simulink model "lab6"  (R2022a)
settings: Solver=FixedStepAuto  StartTime=0.0  StopTime=3  FixedStep=1e-6  MaxStep=1e-5  RelTol=1e-5  EnableMultiTasking=on
undefined symbols (not defined in the file): f_e, I_n, J, km, Lr, Ls, m_f, Pn, Rr, Rs, T_e_rated, T_me_load, U_s, w_ref, zp
libraries: simulink x9, spsFourierLib x6, spsControlledVoltageSourceLib x3, spsAsynchronousMachineSIUnitsLib x2, spsSeriesRLCBranchLib x2, spsThreePhaseVIMeasurementLib x2, spsVoltageMeasurementLib x2, spsUniversalBridgeLib x1, spsDiodeLib x1, spsGroundLib x1, spspowerguiLib x1
settings Model: SimulationMode=accelerator  Creator=Trant  LastModifiedBy=81502
settings SolverCC: AlgebraicLoopSolver=TrustRegion
settings DataIOCC: ReturnWorkspaceOutputs=off
settings DebuggingCC: UnconnectedInputMsg=warning  UnconnectedOutputMsg=warning  UnconnectedLineMsg=warning  SFExecutionAtInitializationDiag=none  SFMachineParentedDataDiag=warning  ArithmeticOperatorsInVariantConditions=warning
settings SFSimCC: SimUseLocalCustomCode=off  CustomCodeUndefinedFunction=UseInterfaceOnly
settings RTWCC: RTWUseLocalCustomCode=off  DLArmComputeVersion=19.05
settings CodeAppCC: StateflowObjectComments=on
settings ConfigComp: CovMetricSettings=dw  CovSaveCumulativeToWorkspaceVar=on  CovSaveSingleToWorkspaceVar=on  CovExternalEMLEnable=off
settings SimscapeCC: SimscapeNormalizeSystem=off

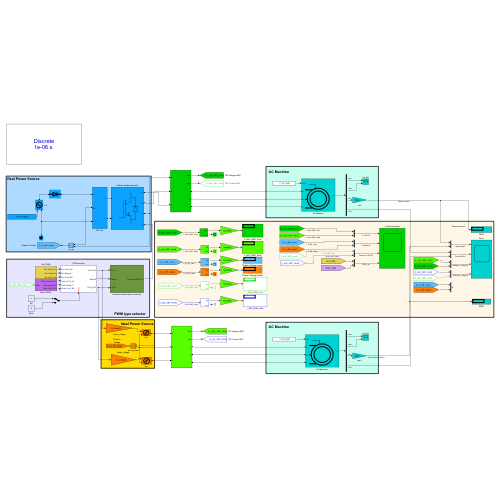
[thumbnail: Simulink's stored preview of the top-level diagram]
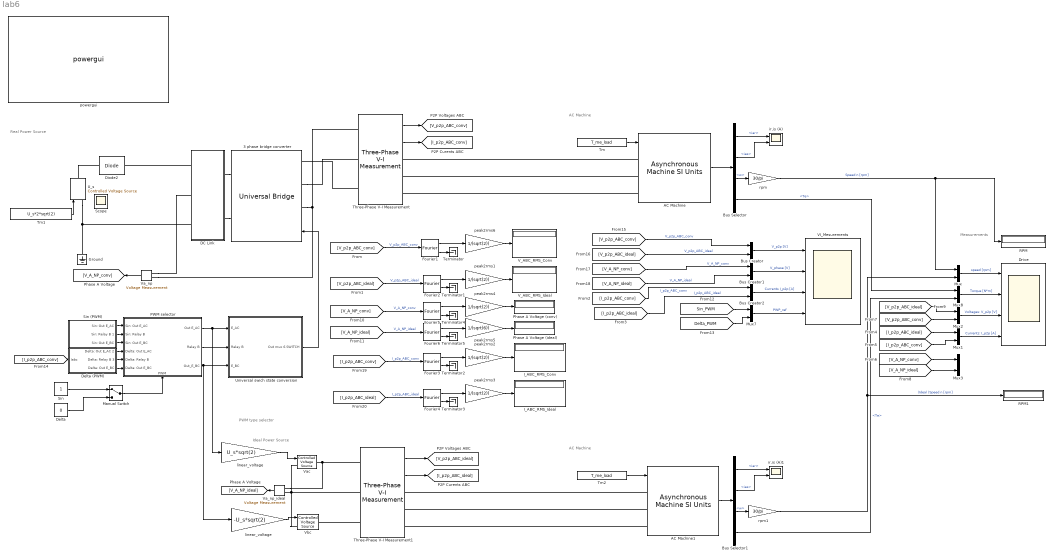
== system lab6 ==
  note: Measurements
  note: Ideal Power Source
  note: Real Power Source
  note: PWM type selector
  note: AC Machine
  note: AC Machine
  3 phase bridge converter : spsUniversalBridgeLib/Universal Bridge  Arms=3  SnubberResistance=1e5  SnubberCapacitance=inf  Device=IGBT / Diodes  Ron=1e-2  Lon=0  ForwardVoltages="[  1.5  0.7  ]"  ForwardVoltage=0  GTOparameters=[ 10e-6 , 20e-6 ]  IGBTparameters=[ 1e-6 , 2e-6 ]  Measurements=None  Measurements_2=None  converterType=Rectifier
  AC Machine : spsAsynchronousMachineSIUnitsLib/Asynchronous Machine SI Units  RotorType=Squirrel-cage  PresetModel=No  MechanicalLoad=Torque Tm  ShowDetailedParameters=on  ReferenceFrame=Stationary  Units=SI  MeasurementBus=on  NominalParameters=[ Pn, U_s*sqrt(3), f_e ]  VoltageRatio=1  Stator="[ Rs  Ls ]"  Rotor="[Rr  Lr ]"  Cage1=[ 0.022 0.226/377]  Cage2=[ 0.022 0.226/377]  Lm=Lm  Mechanical="[ J  0 zp]"  PolePairs=2  InitialConditions="[ 1,0   0,0,0   0,0,0 ]"  SimulateSaturation=off  Saturation=[14.03593122, 27.81365428, 53.79336849, 72.68890987, 97.98006896, 148.6815601, 215.7428561, 302.9841135, 428.7778367 ; 230, 322, 414, 460, 506, 552, 598, 644, 690]  LoadFlowParameters=0  TsPowergui=0  TsBlock=-1  IterativeModel=Trapezoidal non iterative  IterativeDiscreteModel=Trapezoidal non iterative  Pmec=0
      settings: AttributesFormatString=\n
  AC Machine1 : spsAsynchronousMachineSIUnitsLib/Asynchronous Machine SI Units  RotorType=Squirrel-cage  PresetModel=No  MechanicalLoad=Torque Tm  ShowDetailedParameters=on  ReferenceFrame=Stationary  Units=SI  MeasurementBus=on  NominalParameters=[ Pn, U_s*sqrt(3), f_e ]  VoltageRatio=1  Stator="[ Rs  Ls ]"  Rotor="[Rr  Lr ]"  Cage1=[ 0.022 0.226/377]  Cage2=[ 0.022 0.226/377]  Lm=Lm  Mechanical="[ J  0 zp]"  PolePairs=2  InitialConditions="[ 1,0   0,0,0   0,0,0 ]"  SimulateSaturation=off  Saturation=[14.03593122, 27.81365428, 53.79336849, 72.68890987, 97.98006896, 148.6815601, 215.7428561, 302.9841135, 428.7778367 ; 230, 322, 414, 460, 506, 552, 598, 644, 690]  LoadFlowParameters=0  TsPowergui=0  TsBlock=-1  IterativeModel=Trapezoidal non iterative  IterativeDiscreteModel=Trapezoidal non iterative  Pmec=0
      settings: AttributesFormatString=\n
  Bus Creator : BusCreator  Inputs=2
  Bus Creator1 : BusCreator  Inputs=2
  Bus Creator2 : BusCreator  Inputs=2
  Bus Selector : BusSelector  OutputSignals=iar,ias,w,Te
  Bus Selector1 : BusSelector  OutputSignals=iar,ias,w,Te
  DC Link : Subsystem
  Delta : Constant  Value=0
  "Delta (PWM) " : Subsystem
  Diode2 : spsDiodeLib/Diode  Ron=0.0000001  Lon=0  Vf=0.0000001  IC=0  UseSnubber=0  Rs=inf  Cs=250e-9  Measurements=off
  Drive : Scope  NumInputPorts=4
  Fourier{1..6} (6 alike) : spsFourierLib/Fourier  Freq=f_e  n=1  InInit=[0, 0]  Ts=0
      settings: SourceProductBaseCode=PS
  Ground : spsGroundLib/Ground  LConnTagsString=a
  I_ABC_RMS_Conv : Display
      settings: Decimation=100
  I_ABC_RMS_Ideal : Display
      settings: Decimation=100
  Manual Switch : ManualSwitch
  Mux{,1..3,7..8} (6 alike) : Mux  Inputs=2
  PWM selector : Subsystem
      settings: PortSchema="{\"entries\":[{\"content\":{\"sides\":[{\"content\":{\"connectorIds\":[\"In1\",\"In2\",\"In3\",\"In4\",\"In5\",\"In6\"]},\"type\":\"ConnectorPlacement.EquallySpacedRectSide\",\"uuid\":\"d8825297-29c5-47ea-8460-276057c08024\"},{\"content\":{\"connectorIds\":[\"Out1\",\"Out2\",\"Out3\"],\"side\":\"RIGHT\"},\"type\":\"ConnectorPlacement.EquallySpacedRectSide\",\"uuid\":\"df0a2572-9195-4f57-b13e-7b5fffdd47ce\"},{\"content\":{\"connectorIds\":[],\"side\":\"TOP\"},\"type\":\"ConnectorPlacement.EquallySpacedRectSide\",\"uuid\":\"3bcfb922-02d6-49ee-9ecc-d9568c4dbca9\"},{\"content\":{\"connectorIds\":[\"In7\"],\"side\":\"BOTTOM\"},\"type\":\"ConnectorPlacement.EquallySpacedRectSide\",\"uuid\":\"29fdab77-a4c0-4546-9e45-02849de3b5bd\"},{\"content\":{\"connectorIds\":[],\"side\":\"HIDDEN\"},\"type\":\"ConnectorPlacement.EquallySpacedRectSide\",\"uuid\":\"147cb719-0326-42c1-9162-cd1cd750ef12\"}]},\"type\":\"ConnectorPlacement.EquallySpacedConnector\",\"uuid\":\"5ed61148-1717-428a-bdaf-bb7d5a590e8d\"}],\"packageUris\":[\"http://schema.mathworks.com/mf0/Connector/R2020b\"],\"version\":\"1.0\"}"
  Phase A Voltage (conv) : Display
      settings: Decimation=100
  Phase A Voltage (ideal) : Display
      settings: Decimation=100
  RPM : Display
      settings: Decimation=100
  RPM1 : Display
      settings: Decimation=100
  Sin : Constant
  Sin (PWM) : Subsystem
  Terminator{,1..5} (6 alike) : Terminator
  Three-Phase V-I Measurement : spsThreePhaseVIMeasurementLib/Three-Phase V-I Measurement  VoltageMeasurement=phase-to-phase  SetLabelV=off  LabelV=Vabc  Vpu=off  VpuLL=off  CurrentMeasurement=yes  SetLabelI=off  LabelI=Iabc  Ipu=off  Pbase=100e6  Vbase=500e3  OutputType=Complex  PhasorSimulation=off  PSBequivalent=0
  Three-Phase V-I Measurement1 : spsThreePhaseVIMeasurementLib/Three-Phase V-I Measurement  VoltageMeasurement=phase-to-phase  SetLabelV=off  LabelV=Vabc  Vpu=off  VpuLL=off  CurrentMeasurement=yes  SetLabelI=off  LabelI=Iabc  Ipu=off  Pbase=100e6  Vbase=500e3  OutputType=Complex  PhasorSimulation=off  PSBequivalent=0
  Tm : Constant  Value=T_me_load
  Tm1 : Constant  Value=U_s*2*sqrt(2)  VectorParams1D=off
  Tm2 : Constant  Value=T_me_load
  U_s : spsControlledVoltageSourceLib/Controlled Voltage Source  Description=source block  Initialize=on  Source_Type=AC  Amplitude=0  Phase=0  Frequency=0  Measurements=None
      settings: AttributesFormatString=\n
  Universal swich state conversion : Subsystem
  VI_Mesurements : Scope  NumInputPorts=4
  V_ABC_RMS_Conv : Display
      settings: Decimation=100
  V_ABC_RMS_Ideal : Display
      settings: Decimation=100
  Va_np : spsVoltageMeasurementLib/Voltage Measurement  Tag=PoWeRsYsTeMmEaSuReMeNt  PhasorSimulation=off  OutputType=Magnitude  PSBequivalent=0
  Va_np_ideal : spsVoltageMeasurementLib/Voltage Measurement  Tag=PoWeRsYsTeMmEaSuReMeNt  PhasorSimulation=off  OutputType=Magnitude  PSBequivalent=0
  Vac : spsControlledVoltageSourceLib/Controlled Voltage Source  Description=source block  Initialize=on  Source_Type=AC  Amplitude=0  Phase=0  Frequency=0  Measurements=None
      settings: AttributesFormatString=\n
  "Vbc " : spsControlledVoltageSourceLib/Controlled Voltage Source  Description=source block  Initialize=on  Source_Type=AC  Amplitude=0  Phase=0  Frequency=0  Measurements=None
      settings: AttributesFormatString=\n
  ir,is (A) : Scope  NumInputPorts=2
  ir,is (A)1 : Scope  NumInputPorts=2
  linear_voltage : Gain  Gain=U_s*sqrt(2)  SaturateOnIntegerOverflow=on  OutDataTypeStr=Inherit: Same as input  ParamDataTypeStr=Inherit: Same as input
  "linear_voltage " : Gain  Gain=-U_s*sqrt(2)  SaturateOnIntegerOverflow=on  OutDataTypeStr=Inherit: Same as input  ParamDataTypeStr=Inherit: Same as input
  peak2rms{1..4,6} (5 alike) : Gain  Gain=1/(sqrt(2))  SaturateOnIntegerOverflow=on  OutDataTypeStr=Inherit: Same as input  ParamDataTypeStr=Inherit: Same as input
  peak2rms5 : Gain  Gain=1/(sqrt(6))  SaturateOnIntegerOverflow=on  OutDataTypeStr=Inherit: Same as input  ParamDataTypeStr=Inherit: Same as input
  powergui : spspowerguiLib/powergui  SimulationMode=Discrete  SampleTime=1e-6  frequency=60  Iterations=50  frequencyindice=0  Pbase=100e6  ErrMax=1e-4  UnitsV=kV  UnitsW=MW  buscounter=0  FunctionMessages=off  echomessages=off  EnableUseOfTLC=off  CurrentSourceSwitches=on  DisableSnubberDevices=off  DisableRonSwitches=off  DisableVfSwitches=off  DisplayEquations=off  AutomaticDiscreteSolvers=off  SolverType=Tustin/Backward Euler (TBE)  Interpol=off  ExternalGateDelay=off  methode=off  Ts=100  x0status=blocks  SPID=off  SwTol=0  HookPort=off  NonlinearTolerance=1e-4  nMaxIteration=100  ContinueOnMaxIteration=off  RestoreLinks=warning  ResistiveCurrentMeasurement=off  Frange=[0:2:500]  Ylog=off  Xlog=on  ShowGrid=off  save=off  variable=ZData  structure=VI_mesurements  ZoomFFT=off  StartTime=1.55  cycles=1  DisplayStyle=1  fundamental=50  FreqAxis=on  MaxFrequency=40000  frequencyindicesteady=1  RmsSteady=1  display=off
  rpm : Gain  Gain=30/pi  SaturateOnIntegerOverflow=on  OutDataTypeStr=Inherit: Same as input  ParamDataTypeStr=Inherit: Same as input
  rpm1 : Gain  Gain=30/pi  SaturateOnIntegerOverflow=on  OutDataTypeStr=Inherit: Same as input  ParamDataTypeStr=Inherit: Same as input
  Scope : Scope
  wires:
  Tm/1 -> AC Machine/1
  Bus Selector/3 -> rpm/1  "<w>"
  Fourier1/2 -> Terminator/1
  rpm/1 -> Mux/1, RPM/1  "Speed n [rpm]"
  Bus Selector/2 -> ir,is (A)/2  "<ias>"
  peak2rms6/1 -> V_ABC_RMS_Conv/1
  Bus Selector/1 -> ir,is (A)/1  "<iar>"
  AC Machine/1 -> Bus Selector/1
  Fourier1/1 -> peak2rms6/1
  Tm1/1 -> U_s/1
  "linear_voltage "/1 -> "Vbc "/1
  linear_voltage/1 -> Vac/1
  Fourier2/1 -> peak2rms1/1
  Fourier2/2 -> Terminator1/1
  peak2rms1/1 -> V_ABC_RMS_Ideal/1
  Universal swich state conversion/1(Out mux 6 SWITCH) -> 3 phase bridge converter/1
  Manual Switch/1 -> PWM selector/7(PWM)
  Sin/1 -> Manual Switch/1
  Delta/1 -> Manual Switch/2
  Sin (PWM)/1("Sin: Out E_AC ") -> PWM selector/1(Sin: Out E_AC)
  Sin (PWM)/2(Sin: Relay B 1) -> PWM selector/2(Sin: Relay B)
  Sin (PWM)/3(Sin: Out E_BC) -> PWM selector/3(Sin: Out E_BC)
  "Delta (PWM) "/1(Delta: Out E_AC 2) -> PWM selector/4(Delta: Out E_AC)
  "Delta (PWM) "/2(Delta: Relay B 3) -> PWM selector/5(Delta: Relay B)
  "Delta (PWM) "/3(Delta: Out E_BC) -> PWM selector/6(Delta: Out E_BC)
  PWM selector/3(Out_E_BC) -> "linear_voltage "/1, Universal swich state conversion/3(E_BC)
  PWM selector/2(Relay B) -> Universal swich state conversion/2("Relay B ")
  PWM selector/1(Out E_AC) -> Universal swich state conversion/1("E_AC "), linear_voltage/1
  Three-Phase V-I Measurement/1 -> [V_p2p_ABC_conv]
  Three-Phase V-I Measurement1/1 -> [V_p2p_ABC_ideal]
  Three-Phase V-I Measurement1/2 -> [I_p2p_ABC_ideal]
  Three-Phase V-I Measurement/2 -> [I_p2p_ABC_conv]
  [V_p2p_ABC_conv] -> Fourier1/1  "V_p2p_ABC_conv"
  [V_p2p_ABC_ideal] -> Fourier2/1  "V_p2p_ABC_ideal"
  AC Machine1/1 -> Bus Selector1/1
  Tm2/1 -> AC Machine1/1
  Bus Selector1/2 -> ir,is (A)1/2  "<ias>"
  Bus Selector1/1 -> ir,is (A)1/1  "<iar>"
  rpm1/1 -> RPM1/1, Mux/2  "(Ideal )Speed n [rpm]"
  Bus Selector1/3 -> rpm1/1  "<w>"
  Mux/1 -> Drive/1  "speed [rpm]"
  [I_p2p_ABC_ideal] -> Bus Creator2/2  "I_p2p_ABC_ideal"
  [I_p2p_ABC_conv] -> Bus Creator2/1  "I_p2p_ABC_conv"
  peak2rms3/1 -> I_ABC_RMS_Ideal/1
  Fourier4/2 -> Terminator3/1
  Fourier4/1 -> peak2rms3/1
  Fourier3/1 -> peak2rms2/1
  peak2rms2/1 -> I_ABC_RMS_Conv/1
  Fourier3/2 -> Terminator2/1
  [I_p2p_ABC_conv] -> Mux1/2
  [I_p2p_ABC_ideal] -> Mux1/1
  Mux1/1 -> Drive/4  "Currents: I_p2p [A]"
  [V_p2p_ABC_ideal] -> Mux2/1
  [V_p2p_ABC_conv] -> Mux2/2
  Mux2/1 -> Drive/3  "Voltages: V_p2p [V]"
  Va_np/1 -> [V_A_NP_conv]
  Va_np_ideal/1 -> [V_A_NP_ideal]
  [V_A_NP_conv] -> Fourier5/1  "V_A_NP_conv"
  Fourier5/1 -> peak2rms4/1
  peak2rms4/1 -> Phase A Voltage (conv)/1
  Fourier5/2 -> Terminator4/1
  Bus Creator/1 -> VI_Mesurements/1  "V_p2p [V]"
  Bus Creator1/1 -> VI_Mesurements/2  "V_phase [V]"
  Bus Creator2/1 -> VI_Mesurements/3  "Currents I_p2p [A]"
  [Sin_PWM] -> Mux7/1
  [Delta_PWM] -> Mux7/2
  Mux7/1 -> VI_Mesurements/4  "PWP_ref"
  [I_p2p_ABC_conv] -> "Delta (PWM) "/1("Iabc ")
  Fourier6/2 -> Terminator5/1
  peak2rms5/1 -> Phase A Voltage (ideal)/1
  Fourier6/1 -> peak2rms5/1
  Bus Selector/4 -> Mux8/1  "<Te>"
  Bus Selector1/4 -> Mux8/2  "<Te>"
  Mux8/1 -> Drive/2  "Torque [N*m]"
  [V_A_NP_conv] -> Mux3/1
  [V_A_NP_ideal] -> Mux3/2
  [V_A_NP_ideal] -> Fourier6/1  "V_A_NP_ideal"
  [V_p2p_ABC_conv] -> Bus Creator/1  "V_p2p_ABC_conv"
  [V_p2p_ABC_ideal] -> Bus Creator/2  "V_p2p_ABC_ideal"
  [V_A_NP_conv] -> Bus Creator1/1  "V_A_NP_conv"
  [V_A_NP_ideal] -> Bus Creator1/2  "V_A_NP_ideal"
  [I_p2p_ABC_ideal] -> Fourier4/1  "I_p2p_ABC_ideal"
  [I_p2p_ABC_conv] -> Fourier3/1  "I_p2p_ABC_conv"
  connections:
  "Vbc "/LConn1 -- Vac/LConn1 -- Va_np_ideal/LConn2 -- Three-Phase V-I Measurement1/LConn2
  Three-Phase V-I Measurement1/LConn1 -- Va_np_ideal/LConn1 -- Vac/RConn1
  AC Machine/LConn3 -- Three-Phase V-I Measurement/RConn3
  AC Machine/LConn2 -- Three-Phase V-I Measurement/RConn2
  AC Machine/LConn1 -- Three-Phase V-I Measurement/RConn1
  U_s/RConn1 -- Diode2/LConn1
  3 phase bridge converter/LConn2 -- Three-Phase V-I Measurement/LConn2
  Three-Phase V-I Measurement1/LConn3 -- "Vbc "/RConn1
  AC Machine1/LConn1 -- Three-Phase V-I Measurement1/RConn1
  AC Machine1/LConn2 -- Three-Phase V-I Measurement1/RConn2
  AC Machine1/LConn3 -- Three-Phase V-I Measurement1/RConn3
  Three-Phase V-I Measurement/LConn3 -- 3 phase bridge converter/LConn3
  3 phase bridge converter/LConn1 -- Va_np/LConn1 -- Three-Phase V-I Measurement/LConn1
  Ground/LConn1 -- U_s/LConn1 -- DC Link/LConn3
  DC Link/LConn1 -- Diode2/RConn1
  DC Link/RConn2 -- 3 phase bridge converter/RConn1
  DC Link/RConn1 -- 3 phase bridge converter/RConn2
  Va_np/LConn2 -- DC Link/LConn2

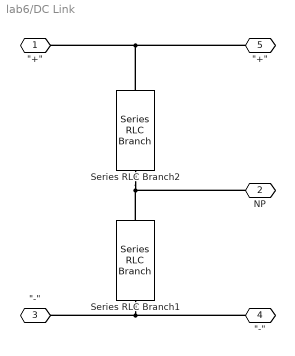
== system lab6/DC Link ==
  Series RLC Branch1 : spsSeriesRLCBranchLib/Series RLC Branch  LConnTagsString=__new0  RConnTagsString=__new0  BranchType=RC  Resistance=0.1  Inductance=1e-3  SetiL0=off  InitialCurrent=0  Capacitance=1e-3  Setx0=off  InitialVoltage=0  Measurements=None
  Series RLC Branch2 : spsSeriesRLCBranchLib/Series RLC Branch  LConnTagsString=__new0  RConnTagsString=__new0  BranchType=RC  Resistance=0.1  Inductance=1e-3  SetiL0=off  InitialCurrent=0  Capacitance=1e-3  Setx0=off  InitialVoltage=0  Measurements=None
  "\"+\"" : PMIOPort  Side=Left
  NP : PMIOPort  Port=2  Side=Left
  "\"-\"" : PMIOPort  Port=3  Side=Left
  "\"-\" " : PMIOPort  Port=4  Side=Right
  "\"+\" " : PMIOPort  Port=5  Side=Right
  connections:
  Series RLC Branch1/LConn1 -- NP/RConn1 -- Series RLC Branch2/RConn1
  Series RLC Branch1/RConn1 -- "\"-\" "/RConn1 -- "\"-\""/RConn1
  Series RLC Branch2/LConn1 -- "\"+\""/RConn1 -- "\"+\" "/RConn1

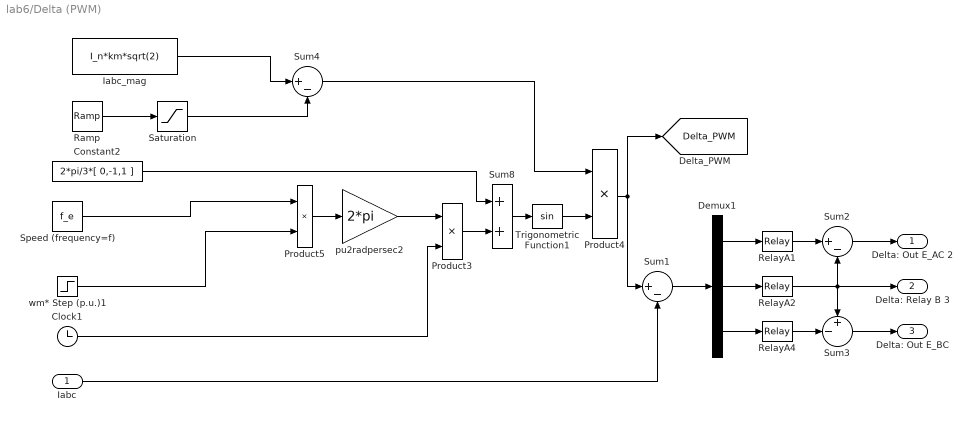
== system lab6/Delta (PWM)  ==
  "Iabc " : Inport
  Clock1 : Clock
  Constant2 : Constant  Value=2*pi/3*[ 0,-1,1 ]
  Demux1 : Demux  Outputs=3
      settings: DisplayOption=none
  Iabc_mag : Constant  Value=I_n*km*sqrt(2)
  Product3 : Product  InputSameDT=on  SaturateOnIntegerOverflow=on  OutDataTypeStr=Inherit: Same as first input
  Product4 : Product  InputSameDT=on  SaturateOnIntegerOverflow=on  OutDataTypeStr=Inherit: Same as first input
  Product5 : Product  InputSameDT=on  SaturateOnIntegerOverflow=on  OutDataTypeStr=Inherit: Same as first input
  Ramp : simulink/Sources/Ramp  slope=1  start=0  InitialOutput=0
  RelayA1 : Relay  OnSwitchValue=0.1  OffSwitchValue=-0.1
  RelayA2 : Relay  OnSwitchValue=0.1  OffSwitchValue=-0.1
  RelayA4 : Relay  OnSwitchValue=0.1  OffSwitchValue=-0.1
  Saturation : Saturate  UpperLimit=T_me_load/T_e_rated*I_n*sqrt(2)  LowerLimit=0
  Speed (frequency=f) : Constant  Value=f_e
  Sum1 : Sum  Inputs=|+-  InputSameDT=on  SaturateOnIntegerOverflow=on  OutDataTypeStr=Inherit: Same as first input
  Sum2 : Sum  Inputs=|+-  InputSameDT=on  SaturateOnIntegerOverflow=on  OutDataTypeStr=Inherit: Same as first input
  Sum3 : Sum  Inputs=+-|  InputSameDT=on  SaturateOnIntegerOverflow=on  OutDataTypeStr=Inherit: Same as first input
  Sum4 : Sum  Inputs=|+-  InputSameDT=on  SaturateOnIntegerOverflow=on  OutDataTypeStr=Inherit: Same as first input
  Sum8 : Sum  InputSameDT=on  SaturateOnIntegerOverflow=on  OutDataTypeStr=Inherit: Same as first input
  Trigonometric Function1 : Trigonometry
  pu2radpersec2 : Gain  Gain=2*pi  SaturateOnIntegerOverflow=on  OutDataTypeStr=Inherit: Same as input  ParamDataTypeStr=Inherit: Same as input
  wm* Step (p.u.)1 : Step  Time=0  After=w_ref  SampleTime=0
  Delta: Out E_AC 2 : Outport  VectorParamsAs1DForOutWhenUnconnected=off
  Delta: Relay B 3 : Outport  Port=2  VectorParamsAs1DForOutWhenUnconnected=off
  Delta: Out E_BC : Outport  Port=3  VectorParamsAs1DForOutWhenUnconnected=off
  tag scope: Delta_PWM=global
  wires:
  Sum3/1 -> Delta: Out E_BC/1
  RelayA2/1 -> Delta: Relay B 3/1, Sum2/2, Sum3/1
  Product5/1 -> pu2radpersec2/1
  Product3/1 -> Sum8/2
  pu2radpersec2/1 -> Product3/1
  RelayA1/1 -> Sum2/1
  Sum2/1 -> Delta: Out E_AC 2/1
  Constant2/1 -> Sum8/1
  Sum8/1 -> Trigonometric Function1/1
  Trigonometric Function1/1 -> Product4/2
  wm* Step (p.u.)1/1 -> Product5/2
  Clock1/1 -> Product3/2
  RelayA4/1 -> Sum3/2
  Speed (frequency=f)/1 -> Product5/1
  Demux1/1 -> RelayA1/1
  Demux1/2 -> RelayA2/1
  Demux1/3 -> RelayA4/1
  Sum1/1 -> Demux1/1
  "Iabc "/1 -> Sum1/2
  Product4/1 -> [Delta_PWM], Sum1/1
  Iabc_mag/1 -> Sum4/1
  Ramp/1 -> Saturation/1
  Saturation/1 -> Sum4/2
  Sum4/1 -> Product4/1

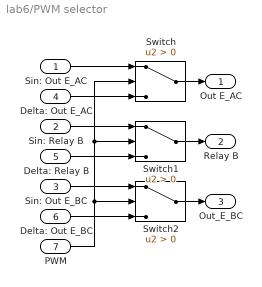
== system lab6/PWM selector ==
  Sin: Out E_AC : Inport
  Sin: Relay B : Inport  Port=2
  Sin: Out E_BC : Inport  Port=3
  Delta: Out E_AC : Inport  Port=4
  Delta: Relay B : Inport  Port=5
  Delta: Out E_BC : Inport  Port=6
  PWM : Inport  Port=7
  Switch : Switch  Criteria=u2 > Threshold  SaturateOnIntegerOverflow=off  InputSameDT=off
  Switch1 : Switch  Criteria=u2 > Threshold  SaturateOnIntegerOverflow=off  InputSameDT=off
  Switch2 : Switch  Criteria=u2 > Threshold  SaturateOnIntegerOverflow=off  InputSameDT=off
  Out E_AC : Outport  VectorParamsAs1DForOutWhenUnconnected=off
  Relay B : Outport  Port=2  VectorParamsAs1DForOutWhenUnconnected=off
  Out_E_BC : Outport  Port=3  VectorParamsAs1DForOutWhenUnconnected=off
  wires:
  Delta: Out E_BC/1 -> Switch2/3
  Sin: Out E_BC/1 -> Switch2/1
  Delta: Relay B/1 -> Switch1/3
  Sin: Relay B/1 -> Switch1/1
  Switch2/1 -> Out_E_BC/1
  Sin: Out E_AC/1 -> Switch/1
  Switch/1 -> Out E_AC/1
  Delta: Out E_AC/1 -> Switch/3
  Switch1/1 -> Relay B/1
  PWM/1 -> Switch/2, Switch1/2, Switch2/2

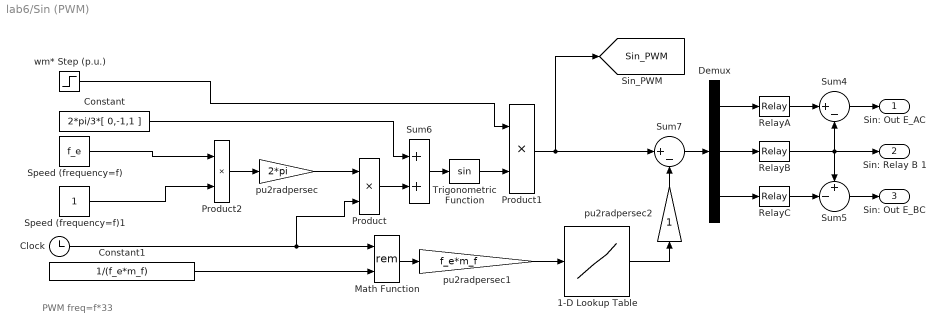
== system lab6/Sin (PWM) ==
  note: PWM freq=f*33
  1-D Lookup Table : Lookup_n-D  NumberOfTableDimensions=1  BreakpointsForDimension1="[0 0.25  0.75  1]"  Table="[0  1  -1  0]"  InternalRulePriority=Speed  RndMeth=Simplest
  Clock : Clock
  Constant : Constant  Value=2*pi/3*[ 0,-1,1 ]
  Constant1 : Constant  Value=1/(f_e*m_f)
  Demux : Demux  Outputs=3
      settings: DisplayOption=none
  Math Function : Math  Operator=rem  SignedPower=on
  Product : Product  InputSameDT=on  SaturateOnIntegerOverflow=on  OutDataTypeStr=Inherit: Same as first input
  Product1 : Product  InputSameDT=on  SaturateOnIntegerOverflow=on  OutDataTypeStr=Inherit: Same as first input
  Product2 : Product  InputSameDT=on  SaturateOnIntegerOverflow=on  OutDataTypeStr=Inherit: Same as first input
  RelayA : Relay  OnSwitchValue=0  OffSwitchValue=0  OffOutputValue=-1
  RelayB : Relay  OnSwitchValue=0  OffSwitchValue=0  OffOutputValue=-1
  RelayC : Relay  OnSwitchValue=0  OffSwitchValue=0  OffOutputValue=-1
  Speed (frequency=f) : Constant  Value=f_e
  Speed (frequency=f)1 : Constant
  Sum4 : Sum  Inputs=|+-  InputSameDT=on  SaturateOnIntegerOverflow=on  OutDataTypeStr=Inherit: Same as first input
  Sum5 : Sum  Inputs=+-|  InputSameDT=on  SaturateOnIntegerOverflow=on  OutDataTypeStr=Inherit: Same as first input
  Sum6 : Sum  InputSameDT=on  SaturateOnIntegerOverflow=on  OutDataTypeStr=Inherit: Same as first input
  Sum7 : Sum  Inputs=|+-  InputSameDT=on  SaturateOnIntegerOverflow=on  OutDataTypeStr=Inherit: Same as first input
  Trigonometric Function : Trigonometry
  pu2radpersec : Gain  Gain=2*pi  SaturateOnIntegerOverflow=on  OutDataTypeStr=Inherit: Same as input  ParamDataTypeStr=Inherit: Same as input
  pu2radpersec1 : Gain  Gain=f_e*m_f  SaturateOnIntegerOverflow=on  OutDataTypeStr=Inherit: Same as input  ParamDataTypeStr=Inherit: Same as input
  pu2radpersec2 : Gain  SaturateOnIntegerOverflow=on  OutDataTypeStr=Inherit: Same as input  ParamDataTypeStr=Inherit: Same as input
  wm* Step (p.u.) : Step  Time=0  After=w_ref  SampleTime=0
  "Sin: Out E_AC " : Outport  VectorParamsAs1DForOutWhenUnconnected=off
  Sin: Relay B 1 : Outport  Port=2  VectorParamsAs1DForOutWhenUnconnected=off
  Sin: Out E_BC : Outport  Port=3  VectorParamsAs1DForOutWhenUnconnected=off
  tag scope: Sin_PWM=global
  wires:
  Speed (frequency=f)/1 -> Product2/1
  Product2/1 -> pu2radpersec/1
  Sum5/1 -> Sin: Out E_BC/1
  Sum4/1 -> "Sin: Out E_AC "/1
  pu2radpersec/1 -> Product/1
  Constant1/1 -> Math Function/2
  Product1/1 -> [Sin_PWM], Sum7/1
  RelayB/1 -> Sin: Relay B 1/1, Sum5/1, Sum4/2
  Sum6/1 -> Trigonometric Function/1
  RelayC/1 -> Sum5/2
  RelayA/1 -> Sum4/1
  wm* Step (p.u.)/1 -> Product1/1
  Clock/1 -> Product/2, Math Function/1
  Demux/2 -> RelayB/1
  Demux/1 -> RelayA/1
  Demux/3 -> RelayC/1
  Product/1 -> Sum6/2
  Constant/1 -> Sum6/1
  Trigonometric Function/1 -> Product1/2
  Sum7/1 -> Demux/1
  Math Function/1 -> pu2radpersec1/1
  1-D Lookup Table/1 -> pu2radpersec2/1
  pu2radpersec1/1 -> 1-D Lookup Table/1
  pu2radpersec2/1 -> Sum7/2
  Speed (frequency=f)1/1 -> Product2/2

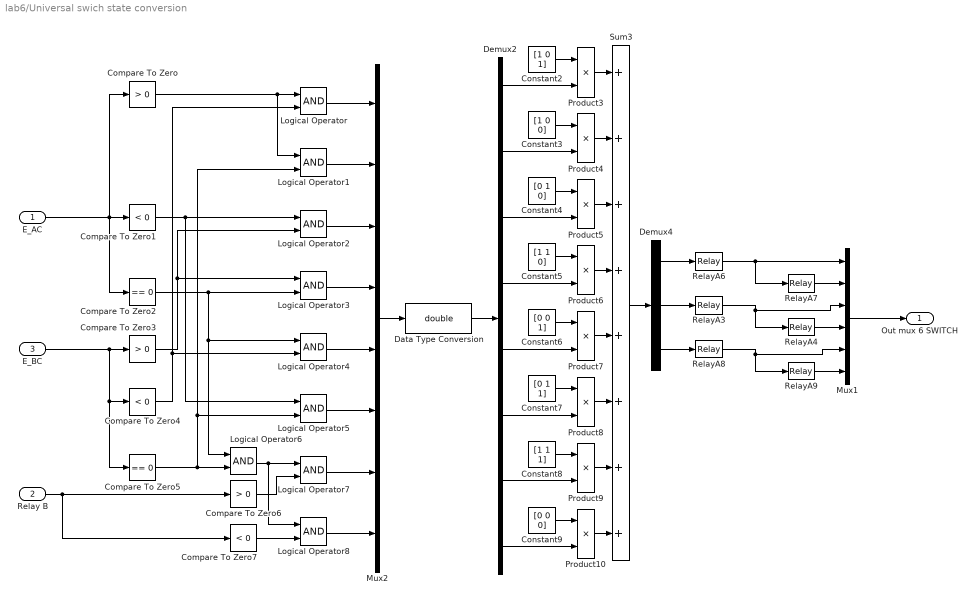
== system lab6/Universal swich state conversion ==
  "E_AC " : Inport
  "Relay B " : Inport  Port=2
  E_BC : Inport  Port=3
  Compare To Zero : simulink/Logic and Bit Operations/Compare To Zero  relop=>  OutDataTypeStr=boolean
  Compare To Zero1 : simulink/Logic and Bit Operations/Compare To Zero  relop=<  OutDataTypeStr=boolean
  Compare To Zero2 : simulink/Logic and Bit Operations/Compare To Zero  relop===  OutDataTypeStr=boolean
  Compare To Zero3 : simulink/Logic and Bit Operations/Compare To Zero  relop=>  OutDataTypeStr=boolean
  Compare To Zero4 : simulink/Logic and Bit Operations/Compare To Zero  relop=<  OutDataTypeStr=boolean
  Compare To Zero5 : simulink/Logic and Bit Operations/Compare To Zero  relop===  OutDataTypeStr=boolean
  Compare To Zero6 : simulink/Logic and Bit Operations/Compare To Zero  relop=>  OutDataTypeStr=boolean
  Compare To Zero7 : simulink/Logic and Bit Operations/Compare To Zero  relop=<  OutDataTypeStr=boolean
  Constant2 : Constant  Value=[1 0 1]
  Constant3 : Constant  Value=[1 0 0]
  Constant4 : Constant  Value="[0 1  0]"
  Constant5 : Constant  Value=[1 1 0]
  Constant6 : Constant  Value=[0 0 1]
  Constant7 : Constant  Value=[0 1 1]
  Constant8 : Constant  Value=[1 1 1]
  Constant9 : Constant  Value=[0 0 0]
  Data Type Conversion : DataTypeConversion  OutDataTypeStr=double  SaturateOnIntegerOverflow=off  RndMeth=Floor
  Demux2 : Demux  Outputs=8
      settings: DisplayOption=none
  Demux4 : Demux  Outputs=3
      settings: DisplayOption=none
  Logical Operator{,1..8} (9 alike) : Logic  AllPortsSameDT=off  OutDataTypeStr=boolean
  Mux1 : Mux  Inputs=6
  Mux2 : Mux  Inputs=8
  Product{3..10} (8 alike) : Product  InputSameDT=on  SaturateOnIntegerOverflow=on  OutDataTypeStr=Inherit: Same as first input
  RelayA3 : Relay  OnSwitchValue=0.02  OffSwitchValue=0.01
  RelayA4 : Relay  OnSwitchValue=0.02  OffSwitchValue=0.01  OnOutputValue=0  OffOutputValue=1
  RelayA6 : Relay  OnSwitchValue=0.02  OffSwitchValue=0.01
  RelayA7 : Relay  OnSwitchValue=0.02  OffSwitchValue=0.01  OnOutputValue=0  OffOutputValue=1
  RelayA8 : Relay  OnSwitchValue=0.02  OffSwitchValue=0.01
  RelayA9 : Relay  OnSwitchValue=0.02  OffSwitchValue=0.01  OnOutputValue=0  OffOutputValue=1
  Sum3 : Sum  Inputs=++++++++  InputSameDT=on  SaturateOnIntegerOverflow=on  OutDataTypeStr=Inherit: Same as first input
  Out mux 6 SWITCH : Outport  VectorParamsAs1DForOutWhenUnconnected=off
  wires:
  Constant2/1 -> Product3/1
  Constant3/1 -> Product4/1
  Demux2/1 -> Product3/2
  Demux2/6 -> Product8/2
  Demux2/5 -> Product7/2
  Constant4/1 -> Product5/1
  Product8/1 -> Sum3/6
  Product10/1 -> Sum3/8
  Product6/1 -> Sum3/4
  Demux2/4 -> Product6/2
  Demux2/3 -> Product5/2
  Demux2/2 -> Product4/2
  Constant6/1 -> Product7/1
  RelayA3/1 -> Mux1/3, RelayA4/1
  RelayA4/1 -> Mux1/4
  Demux4/2 -> RelayA3/1
  RelayA8/1 -> Mux1/5, RelayA9/1
  Demux4/3 -> RelayA8/1
  RelayA9/1 -> Mux1/6
  Demux2/8 -> Product10/2
  Constant7/1 -> Product8/1
  Product3/1 -> Sum3/1
  Product4/1 -> Sum3/2
  Constant5/1 -> Product6/1
  RelayA7/1 -> Mux1/2
  RelayA6/1 -> RelayA7/1, Mux1/1
  Sum3/1 -> Demux4/1
  Mux1/1 -> Out mux 6 SWITCH/1
  Demux4/1 -> RelayA6/1
  Demux2/7 -> Product9/2
  Constant9/1 -> Product10/1
  Product5/1 -> Sum3/3
  Product9/1 -> Sum3/7
  Product7/1 -> Sum3/5
  Constant8/1 -> Product9/1
  Compare To Zero1/1 -> Logical Operator5/1, Logical Operator2/1
  Logical Operator5/1 -> Mux2/6
  Compare To Zero3/1 -> Logical Operator2/2, Logical Operator3/1
  Logical Operator6/1 -> Logical Operator8/1, Logical Operator7/1
  Mux2/1 -> Data Type Conversion/1
  Compare To Zero7/1 -> Logical Operator8/2
  Compare To Zero5/1 -> Logical Operator1/2, Logical Operator5/2, Logical Operator6/2
  Logical Operator8/1 -> Mux2/8
  Compare To Zero2/1 -> Logical Operator3/2, Logical Operator4/1, Logical Operator6/1
  Compare To Zero/1 -> Logical Operator1/1, Logical Operator/1
  "E_AC "/1 -> Compare To Zero1/1, Compare To Zero2/1, Compare To Zero/1
  "Relay B "/1 -> Compare To Zero7/1, Compare To Zero6/1
  Compare To Zero6/1 -> Logical Operator7/2
  Compare To Zero4/1 -> Logical Operator/2, Logical Operator4/2
  Logical Operator1/1 -> Mux2/2
  Logical Operator2/1 -> Mux2/3
  E_BC/1 -> Compare To Zero4/1, Compare To Zero5/1, Compare To Zero3/1
  Logical Operator4/1 -> Mux2/5
  Logical Operator3/1 -> Mux2/4
  Logical Operator7/1 -> Mux2/7
  Logical Operator/1 -> Mux2/1
  Data Type Conversion/1 -> Demux2/1
